simulink model "PowerPlant_Unit"  (R2021a)
settings: Solver=ode23t  StartTime=0.0  StopTime=20  RelTol=1e-3  AbsTol=1e-3
libraries: nesl_utility x15, fl_lib x13, ee_lib x9
settings Model: PacingRate=1000  Creator=ykamatan  LastModifiedBy=ykamatan
settings SolverCC: AutoScaleAbsTol=off  SolverJacobianMethodControl=SparsePerturbation  DaesscMode=Fast
settings DataIOCC: SaveOutput=off  SaveTime=off
settings DebuggingCC: SymbolicDimsDataTypeCodeGenerationDiagnostic=none  SFMachineParentedDataDiag=warning
settings SFSimCC: CustomCodeUndefinedFunction=UseInterfaceOnly
settings SimscapeCC: SimscapeLogSimulationStatistics=on  SimscapeLogDataHistory=10000

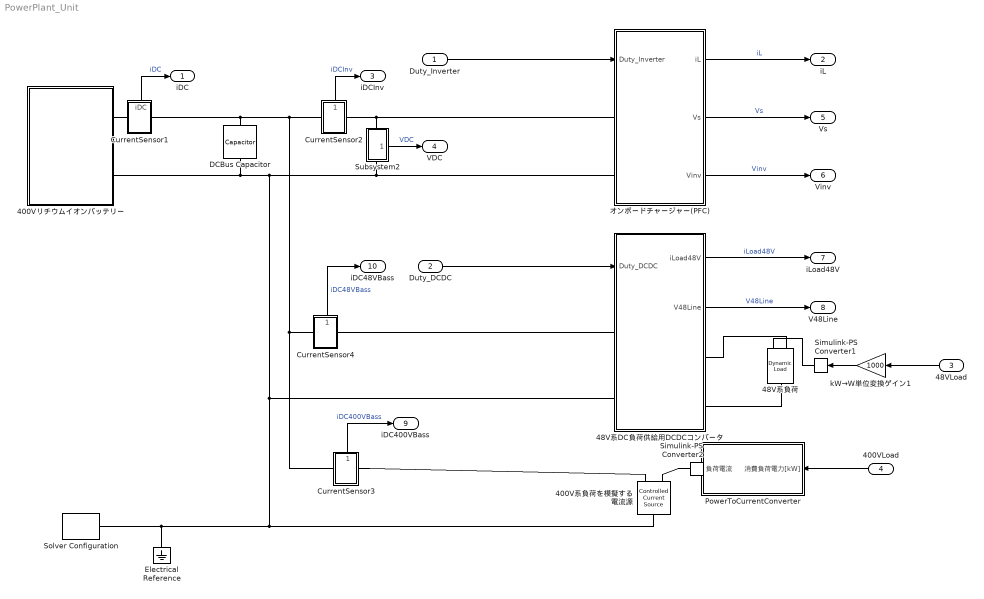
== system PowerPlant_Unit ==
  Duty_Inverter : Inport  OutDataTypeStr=double  PortDimensions=1  SampleTime=0
  Duty_DCDC : Inport  Port=2  OutDataTypeStr=double  PortDimensions=1  SampleTime=0
  48VLoad : Inport  Port=3
  400VLoad : Inport  Port=4
  400Vリチウムイオンバッテリー : Subsystem
  400V系負荷を模擬する 電流源 : fl_lib/Electrical/Electrical Sources/Controlled Current Source
  48V系DC負荷供給用DCDCコンバータ : Subsystem
  48V系負荷 : ee_lib/Passive/Dynamic Load  load_type=ee.enum.dc_ac.dc  enable_fault=ee.enum.faults.faultEnable.no  min_supply_voltage=38 V  pow_min=1e-3 W  G_reverse=1e-6 S  deltaV=1e-3 V  f0=60 Hz  Vrms_min=200 V  Pmin=1e-3 W  fault_action=ee.enum.faults.faultAction.none  t_fault=1 s  open_conductance=1e-4 S
      settings: SourceProductBaseCode=PS  InternalSimscapePortConfiguration="{\"Bottom\":[],\"Left\":[{\"id\":\"p\",\"label\":\"+\",\"type\":\"foundation.electrical.electrical\"}],\"Right\":[{\"id\":\"n\",\"label\":\"-\",\"type\":\"foundation.electrical.electrical\"}],\"Top\":[{\"id\":\"P\",\"label\":\"P\",\"type\":\"input\"}]}"
  CurrentSensor1 : Subsystem
      settings: PortSchema="{\"entries\":[{\"content\":{\"sides\":[{\"content\":{\"connectorIds\":[\"LConn1\"]},\"type\":\"ConnectorPlacement.EquallySpacedRectSide\",\"uuid\":\"7286f59e-cee0-499d-832c-cf6f33a1b017\"},{\"content\":{\"connectorIds\":[\"RConn1\"],\"side\":\"RIGHT\"},\"type\":\"ConnectorPlacement.EquallySpacedRectSide\",\"uuid\":\"6a983281-a6bc-4a57-a5ba-c4da9a8828f4\"},{\"content\":{\"connectorIds\":[\"Out1\"],\"side\":\"TOP\"},\"type\":\"ConnectorPlacement.EquallySpacedRectSide\",\"uuid\":\"6969f7e7-2dce-4d64-b6f6-e92ef9035b1a\"}]},\"type\":\"ConnectorPlacement.EquallySpacedConnector\",\"uuid\":\"05fc616a-5402-4b75-b59e-8cf259d71f3d\"}],\"packageUris\":[\"http://schema.mathworks.com/mf0/Connector/R2020b\"],\"version\":\"1.0\"}"
  CurrentSensor2 : Subsystem
      settings: PortSchema="{\"entries\":[{\"content\":{\"sides\":[{\"content\":{\"connectorIds\":[\"LConn1\"]},\"type\":\"ConnectorPlacement.EquallySpacedRectSide\",\"uuid\":\"7286f59e-cee0-499d-832c-cf6f33a1b017\"},{\"content\":{\"connectorIds\":[\"RConn1\"],\"side\":\"RIGHT\"},\"type\":\"ConnectorPlacement.EquallySpacedRectSide\",\"uuid\":\"6a983281-a6bc-4a57-a5ba-c4da9a8828f4\"},{\"content\":{\"connectorIds\":[\"Out1\"],\"side\":\"TOP\"},\"type\":\"ConnectorPlacement.EquallySpacedRectSide\",\"uuid\":\"6969f7e7-2dce-4d64-b6f6-e92ef9035b1a\"}]},\"type\":\"ConnectorPlacement.EquallySpacedConnector\",\"uuid\":\"05fc616a-5402-4b75-b59e-8cf259d71f3d\"}],\"packageUris\":[\"http://schema.mathworks.com/mf0/Connector/R2020b\"],\"version\":\"1.0\"}"
  CurrentSensor3 : Subsystem
      settings: PortSchema="{\"entries\":[{\"content\":{\"sides\":[{\"content\":{\"connectorIds\":[\"LConn1\"]},\"type\":\"ConnectorPlacement.EquallySpacedRectSide\",\"uuid\":\"7286f59e-cee0-499d-832c-cf6f33a1b017\"},{\"content\":{\"connectorIds\":[\"RConn1\"],\"side\":\"RIGHT\"},\"type\":\"ConnectorPlacement.EquallySpacedRectSide\",\"uuid\":\"6a983281-a6bc-4a57-a5ba-c4da9a8828f4\"},{\"content\":{\"connectorIds\":[\"Out1\"],\"side\":\"TOP\"},\"type\":\"ConnectorPlacement.EquallySpacedRectSide\",\"uuid\":\"6969f7e7-2dce-4d64-b6f6-e92ef9035b1a\"}]},\"type\":\"ConnectorPlacement.EquallySpacedConnector\",\"uuid\":\"05fc616a-5402-4b75-b59e-8cf259d71f3d\"}],\"packageUris\":[\"http://schema.mathworks.com/mf0/Connector/R2020b\"],\"version\":\"1.0\"}"
  CurrentSensor4 : Subsystem
      settings: PortSchema="{\"entries\":[{\"content\":{\"sides\":[{\"content\":{\"connectorIds\":[\"LConn1\"]},\"type\":\"ConnectorPlacement.EquallySpacedRectSide\",\"uuid\":\"7286f59e-cee0-499d-832c-cf6f33a1b017\"},{\"content\":{\"connectorIds\":[\"RConn1\"],\"side\":\"RIGHT\"},\"type\":\"ConnectorPlacement.EquallySpacedRectSide\",\"uuid\":\"6a983281-a6bc-4a57-a5ba-c4da9a8828f4\"},{\"content\":{\"connectorIds\":[\"Out1\"],\"side\":\"TOP\"},\"type\":\"ConnectorPlacement.EquallySpacedRectSide\",\"uuid\":\"6969f7e7-2dce-4d64-b6f6-e92ef9035b1a\"}]},\"type\":\"ConnectorPlacement.EquallySpacedConnector\",\"uuid\":\"05fc616a-5402-4b75-b59e-8cf259d71f3d\"}],\"packageUris\":[\"http://schema.mathworks.com/mf0/Connector/R2020b\"],\"version\":\"1.0\"}"
  DCBus Capacitor : ee_lib/Passive/Capacitor  cap_option=0  c=1000e-6 F  Cvec=[1e-05, 1e-06] F  Vvec=[0, 10] V  CV_table_symmetry=1  f_vec=[1, 10] kHz  DFext_vec=[.8, 1.2]  C_tol=5  enable_C_tol=0  tol_distribution=1  nSigma=4  r=1e-6 Ohm  g=0 1/Ohm  averaging_period=0 s  enable_operating_limits=0  operating_limit_action=2  max_working_voltage_range=[-25, 25] V  power_rating=1 W  enable_faults=0  fault_action=1  Cscale_faulted=100  R_faulted=1e-3 Ohm  G_faulted=0 1/Ohm  tau_fault=1e-3 s  enable_temporal_fault=0  t_fault=1 s  enable_behavioral_fault=0  max_permissible_voltage_range=[-100, 100] V  t_fail_on_voltage=1 s  i_specify=off  i_priority=None  i=0 A  i_nominal_specify=off  i_nominal_unit=A  i_nominal_value=1  v_specify=off  v_priority=None  v=400 V  v_nominal_specify=off  v_nominal_unit=V  v_nominal_value=1  vc_specify=on  vc_priority=High  vc=400 V  vc_nominal_specify=off  vc_nominal_unit=V  vc_nominal_value=1
  Electrical Reference : fl_lib/Electrical/Electrical Elements/Electrical Reference
  PowerToCurrentConverter : Subsystem
  Simulink-PS Converter1 : nesl_utility/Simulink-PS Converter  PhysicalDomain=network_engine_domain  SubClassName=ps_input  LeftPortType=input  RightPortType=output  PseudoPeriodic=off  Frequencies=[]  NoiseDistribution=none  NoiseParameters=[]  Unit=1  AffineConversion=off  FilteringAndDerivatives=provide  SimscapeFilterOrder=1  InputFilterTimeConstant=0.001  UdotUserProvided=0
      settings: SourceProductBaseCode=PW,SS
  Simulink-PS Converter2 : nesl_utility/Simulink-PS Converter  PhysicalDomain=network_engine_domain  SubClassName=ps_input  LeftPortType=input  RightPortType=output  PseudoPeriodic=off  Frequencies=[]  NoiseDistribution=none  NoiseParameters=[]  Unit=1  AffineConversion=off  FilteringAndDerivatives=provide  SimscapeFilterOrder=1  InputFilterTimeConstant=0.001  UdotUserProvided=0
      settings: SourceProductBaseCode=PW,SS
  Solver Configuration : nesl_utility/Solver Configuration  PhysicalDomain=network_engine_domain  SubClassName=solver  LeftPortType=input  RightPortType=generic  Tones=[]  Harmonics=[]  SimulateNoise=off  Profile=off  UseLocalSampling=off  EnableSwitchedLinearOptims=on  FrequencyDomain=off  UseCCode=off  RelTol=0.001  AbsTol=1e-06  MinStep=1e-09  ToWorkspace=off  RevertToSquareIcSolve=off  NumHomotopyIterations=100  PhasorMode=off  PhasorModeNumHarmonics=1  DoDC=off  ResidualTolerance=1e-09  UseLocalSolver=off  LocalSolverChoice=NE_BACKWARD_EULER_ADVANCER  LocalSolverSampleTime=0.001  DoFixedCost=off  MaxNonlinIter=3  MaxModeIter=2  ComputeImpulses=off  ImpulseIterations=2  LinearAlgebra=auto  EquationFormulation=NE_TIME_EF  DelaysMemoryBudget=1024  AutomaticFiltering=on  FilteringTimeConstant=0.001  PartitionStorageMethod=AS_NEEDED  PartitionMemoryBudget=1024  PartitionMethod=ROBUST
      settings: SourceProductBaseCode=PW,SS
  Subsystem2 : Subsystem
      settings: PortSchema="{\"entries\":[{\"content\":{\"sides\":[{\"content\":{\"connectorIds\":[\"Out1\"]},\"type\":\"ConnectorPlacement.EquallySpacedRectSide\",\"uuid\":\"7286f59e-cee0-499d-832c-cf6f33a1b017\"},{\"content\":{\"connectorIds\":[],\"side\":\"RIGHT\"},\"type\":\"ConnectorPlacement.EquallySpacedRectSide\",\"uuid\":\"6a983281-a6bc-4a57-a5ba-c4da9a8828f4\"},{\"content\":{\"connectorIds\":[\"LConn1\"],\"side\":\"TOP\"},\"type\":\"ConnectorPlacement.EquallySpacedRectSide\",\"uuid\":\"6969f7e7-2dce-4d64-b6f6-e92ef9035b1a\"},{\"content\":{\"connectorIds\":[\"RConn1\"],\"side\":\"BOTTOM\"},\"type\":\"ConnectorPlacement.EquallySpacedRectSide\",\"uuid\":\"8f7d22cd-967a-487e-912d-7270502758f1\"}]},\"type\":\"ConnectorPlacement.EquallySpacedConnector\",\"uuid\":\"05fc616a-5402-4b75-b59e-8cf259d71f3d\"}],\"packageUris\":[\"http://schema.mathworks.com/mf0/Connector/R2020b\"],\"version\":\"1.0\"}"
  kW→W単位変換ゲイン1 : Gain  Gain=1000
  オンボードチャージャー(PFC) : Subsystem
  iDC : Outport  OutDataTypeStr=double  PortDimensions=1  SampleTime=0
  iL : Outport  Port=2  OutDataTypeStr=double  PortDimensions=1  SampleTime=0
  iDCInv : Outport  Port=3  OutDataTypeStr=double  PortDimensions=1  SampleTime=0
  VDC : Outport  Port=4  OutDataTypeStr=double  PortDimensions=1  SampleTime=0
  Vs : Outport  Port=5  OutDataTypeStr=double  PortDimensions=1  SampleTime=0
  Vinv : Outport  Port=6  OutDataTypeStr=double  PortDimensions=1  SampleTime=0
  iLoad48V : Outport  Port=7  OutDataTypeStr=double  PortDimensions=1  SampleTime=0
  V48Line : Outport  Port=8  OutDataTypeStr=double  PortDimensions=1  SampleTime=0
  iDC400VBass : Outport  Port=9  OutDataTypeStr=double  PortDimensions=1  SampleTime=0
  iDC48VBass : Outport  Port=10  OutDataTypeStr=double  PortDimensions=1  SampleTime=0
  wires:
  48V系DC負荷供給用DCDCコンバータ/1(iLoad48V) -> iLoad48V/1  "iLoad48V"
  オンボードチャージャー(PFC)/3(Vinv) -> Vinv/1  "Vinv"
  CurrentSensor2/1(iDCInv) -> iDCInv/1  "iDCInv"
  48V系DC負荷供給用DCDCコンバータ/2(V48Line) -> V48Line/1  "V48Line"
  CurrentSensor1/1(iDC) -> iDC/1  "iDC"
  オンボードチャージャー(PFC)/2(Vs) -> Vs/1  "Vs"
  PowerToCurrentConverter/1(負荷電流) -> Simulink-PS Converter2/1
  400VLoad/1 -> PowerToCurrentConverter/1(消費負荷電力[kW])
  CurrentSensor3/1(iDC400VBass) -> iDC400VBass/1  "iDC400VBass"
  kW→W単位変換ゲイン1/1 -> Simulink-PS Converter1/1
  48VLoad/1 -> kW→W単位変換ゲイン1/1
  Subsystem2/1(Vdc) -> VDC/1  "VDC"
  Duty_Inverter/1 -> オンボードチャージャー(PFC)/1(Duty_Inverter)
  CurrentSensor4/1(iDC48VBass) -> iDC48VBass/1  "iDC48VBass"
  オンボードチャージャー(PFC)/1(iL) -> iL/1  "iL"
  Duty_DCDC/1 -> 48V系DC負荷供給用DCDCコンバータ/1(Duty_DCDC)
  connections:
  400Vリチウムイオンバッテリー/RConn2 -- DCBus Capacitor/RConn1 -- Solver Configuration/RConn1 -- Electrical Reference/LConn1 -- 400V系負荷を模擬する 電流源/LConn1 -- 48V系DC負荷供給用DCDCコンバータ/LConn2 -- Subsystem2/RConn1 -- オンボードチャージャー(PFC)/LConn2
  Subsystem2/LConn1 -- CurrentSensor2/RConn1 -- オンボードチャージャー(PFC)/LConn1
  CurrentSensor2/LConn1 -- CurrentSensor3/LConn1 -- CurrentSensor4/LConn1 -- DCBus Capacitor/LConn1 -- CurrentSensor1/RConn1
  Simulink-PS Converter2/RConn1 -- 400V系負荷を模擬する 電流源/RConn1
  CurrentSensor1/LConn1 -- 400Vリチウムイオンバッテリー/RConn1
  48V系負荷/RConn1 -- 48V系DC負荷供給用DCDCコンバータ/RConn2
  48V系DC負荷供給用DCDCコンバータ/RConn1 -- 48V系負荷/LConn1
  Simulink-PS Converter1/RConn1 -- 48V系負荷/LConn2
  CurrentSensor3/RConn1 -- 400V系負荷を模擬する 電流源/RConn2
  CurrentSensor4/RConn1 -- 48V系DC負荷供給用DCDCコンバータ/LConn1

== system PowerPlant_Unit/400Vリチウムイオンバッテリー ==
  400V 理想特性蓄電池 : ee_lib/Sources/Battery  Vnom=400 V  prm_dir=1  R1_dis=2 Ohm  R1_ch=2 Ohm  R1=1 Ohm  prm_AH=2  AH=0.5 hr*A  V1=380 V  AH1=0.25 hr*A  prm_R2=1  R2=2000 Ohm  prm_dyn=2  Rp1=0.05 Ohm  tau1=30 s  Rp2=0.005 Ohm  tau2=30 s  Rp3=0.005 Ohm  tau3=30 s  Rp4=0.005 Ohm  tau4=30 s  Rp5=0.005 Ohm  tau5=30 s  prm_fade=1  N_fade=100  AH_fade=45 hr*A  R1_fade=2.02 Ohm  R1_ch_fade=2.02 Ohm  V1_fade=10.35 V  prm_age=1  prm_age_OCV=1  OCV_age=0.9  SOC_age=60  Tmeas_age=298.15 K  delta_time_age_vec=[0] d  temperature_age_vec=[273] K  OCV_scaling_age=2.2134e6  OCV_offset_age=1.632e6  temp_exp_age=0.515833569 V  t_exp_age=0.75  i_specify=off  i_priority=None  i=0 A  i_nominal_specify=off  i_nominal_unit=A  i_nominal_value=1  v_specify=off  v_priority=None  v=0 V  v_nominal_specify=off  v_nominal_unit=V  v_nominal_value=1  charge_specify=on  charge_priority=High  charge=0.25 hr*A  charge_nominal_specify=off  charge_nominal_unit=hr*A  charge_nominal_value=1  num_cycles_specify=off  num_cycles_priority=High  num_cycles=0  num_cycles_nominal_specify=off  num_cycles_nominal_unit=1  num_cycles_nominal_value=1  thermal_mass=30000 J/K  Tmeas=298.15 K  Vnom_T2=12 V  R1_T2=2.2 Ohm  R1_T2_dis=2.2 Ohm  R1_T2_ch=2.2 Ohm  V1_T2=11.4 V  R2_T2=2200 Ohm  Rp1_T2=0.005 Ohm  tau1_T2=30 s  Rp2_T2=0.005 Ohm  tau2_T2=30 s  Rp3_T2=0.005 Ohm  tau3_T2=30 s  Rp4_T2=0.005 Ohm  tau4_T2=30 s  Rp5_T2=0.005 Ohm  tau5_T2=30 s  Tmeas2=273.15 K  temperature_specify=off  temperature_priority=High  temperature=298.15 K  temperature_nominal_specify=off  temperature_nominal_unit=K  temperature_nominal_value=1
  Bat+ : PMIOPort  Side=Right
  Bat- : PMIOPort  Port=2  Side=Right
  connections:
  400V 理想特性蓄電池/RConn1 -- Bat-/RConn1
  Bat+/RConn1 -- 400V 理想特性蓄電池/LConn1

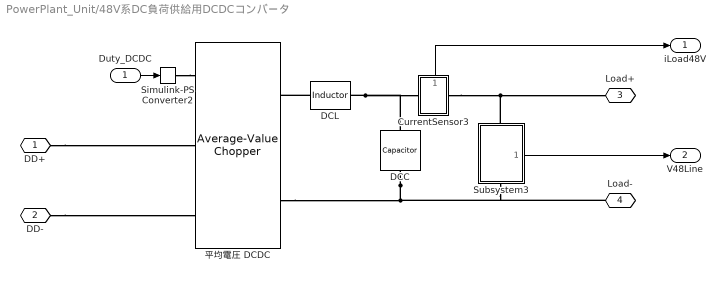
== system PowerPlant_Unit/48V系DC負荷供給用DCDCコンバータ ==
  Duty_DCDC : Inport
  CurrentSensor3 : Subsystem
      settings: PortSchema="{\"entries\":[{\"content\":{\"sides\":[{\"content\":{\"connectorIds\":[\"LConn1\"]},\"type\":\"ConnectorPlacement.EquallySpacedRectSide\",\"uuid\":\"7286f59e-cee0-499d-832c-cf6f33a1b017\"},{\"content\":{\"connectorIds\":[\"RConn1\"],\"side\":\"RIGHT\"},\"type\":\"ConnectorPlacement.EquallySpacedRectSide\",\"uuid\":\"6a983281-a6bc-4a57-a5ba-c4da9a8828f4\"},{\"content\":{\"connectorIds\":[\"Out1\"],\"side\":\"TOP\"},\"type\":\"ConnectorPlacement.EquallySpacedRectSide\",\"uuid\":\"6969f7e7-2dce-4d64-b6f6-e92ef9035b1a\"}]},\"type\":\"ConnectorPlacement.EquallySpacedConnector\",\"uuid\":\"05fc616a-5402-4b75-b59e-8cf259d71f3d\"}],\"packageUris\":[\"http://schema.mathworks.com/mf0/Connector/R2020b\"],\"version\":\"1.0\"}"
  DCC : ee_lib/Passive/Capacitor  cap_option=0  c=100e-6 F  Cvec=[1e-05, 1e-06] F  Vvec=[0, 10] V  CV_table_symmetry=1  f_vec=[1, 10] kHz  DFext_vec=[.8, 1.2]  C_tol=5  enable_C_tol=0  tol_distribution=1  nSigma=4  r=100e-3 Ohm  g=0 1/Ohm  averaging_period=0 s  enable_operating_limits=0  operating_limit_action=2  max_working_voltage_range=[-25, 25] V  power_rating=1 W  enable_faults=0  fault_action=1  Cscale_faulted=100  R_faulted=1e-3 Ohm  G_faulted=0 1/Ohm  tau_fault=1e-3 s  enable_temporal_fault=0  t_fault=1 s  enable_behavioral_fault=0  max_permissible_voltage_range=[-100, 100] V  t_fail_on_voltage=1 s  i_specify=off  i_priority=None  i=0 A  i_nominal_specify=off  i_nominal_unit=A  i_nominal_value=1  v_specify=off  v_priority=None  v=400 V  v_nominal_specify=off  v_nominal_unit=V  v_nominal_value=1  vc_specify=on  vc_priority=High  vc=48 V  vc_nominal_specify=off  vc_nominal_unit=V  vc_nominal_value=1
  DCL : ee_lib/Passive/Inductor  l=10e-6 H  L_tol=20  enable_L_tol=0  tol_distribution=1  nSigma=4  r=0.1 Ohm  g=1e-9 1/Ohm  enable_operating_limits=0  operating_limit_action=2  max_working_current=1 A  power_rating=1 W  enable_faults=0  fault_action=1  lambdaPercent=50  k_faulted=0.9999  turnsShort=0  openCct=0  groundShort=0  groundShortG=0 1/Ohm  tau_fault=1e-3 s  enable_temporal_fault=0  t_fault=1 s  enable_behavioral_fault=0  max_permissible_voltage=100 V  n_fail_on_voltage=1  max_permissible_current=1 A  t_fail_on_current=1 s  i_L_specify=off  i_L_priority=High  i_L=0 A  i_L_nominal_specify=off  i_L_nominal_unit=A  i_L_nominal_value=1
  Simulink-PS Converter2 : nesl_utility/Simulink-PS Converter  PhysicalDomain=network_engine_domain  SubClassName=ps_input  LeftPortType=input  RightPortType=output  PseudoPeriodic=off  Frequencies=[]  NoiseDistribution=none  NoiseParameters=[]  Unit=1  AffineConversion=off  FilteringAndDerivatives=provide  SimscapeFilterOrder=1  InputFilterTimeConstant=0.001  UdotUserProvided=0
      settings: SourceProductBaseCode=PW,SS
  Subsystem3 : Subsystem
      settings: PortSchema="{\"entries\":[{\"content\":{\"sides\":[{\"content\":{\"connectorIds\":[]},\"type\":\"ConnectorPlacement.EquallySpacedRectSide\",\"uuid\":\"7286f59e-cee0-499d-832c-cf6f33a1b017\"},{\"content\":{\"connectorIds\":[\"Out1\"],\"side\":\"RIGHT\"},\"type\":\"ConnectorPlacement.EquallySpacedRectSide\",\"uuid\":\"6a983281-a6bc-4a57-a5ba-c4da9a8828f4\"},{\"content\":{\"connectorIds\":[\"LConn1\"],\"side\":\"TOP\"},\"type\":\"ConnectorPlacement.EquallySpacedRectSide\",\"uuid\":\"6969f7e7-2dce-4d64-b6f6-e92ef9035b1a\"},{\"content\":{\"connectorIds\":[\"RConn1\"],\"side\":\"BOTTOM\"},\"type\":\"ConnectorPlacement.EquallySpacedRectSide\",\"uuid\":\"8f7d22cd-967a-487e-912d-7270502758f1\"}]},\"type\":\"ConnectorPlacement.EquallySpacedConnector\",\"uuid\":\"05fc616a-5402-4b75-b59e-8cf259d71f3d\"}],\"packageUris\":[\"http://schema.mathworks.com/mf0/Connector/R2020b\"],\"version\":\"1.0\"}"
  平均電圧 DCDC : ee_lib/Semiconductors & Converters/Converters/Average-Value Chopper  chopper_type=5  efficiency_option=1  efficiency_fixed=100  i_vec=[0, 2, 5] A  efficiency_vec=[90, 95, 98]
      settings: SourceProductBaseCode=PS  InternalSimscapePortConfiguration="{\"Bottom\":[],\"Left\":[{\"id\":\"DutyCycle\",\"label\":\"DutyCycle\",\"type\":\"input\"},{\"id\":\"p1\",\"label\":\"1+\",\"type\":\"foundation.electrical.electrical\"},{\"id\":\"n1\",\"label\":\"1-\",\"type\":\"foundation.electrical.electrical\"}],\"Right\":[{\"id\":\"p2\",\"label\":\"2+\",\"type\":\"foundation.electrical.electrical\"},{\"id\":\"n2\",\"label\":\"2-\",\"type\":\"foundation.electrical.electrical\"}],\"Top\":[]}"
  DD+ : PMIOPort  Side=Left
  DD- : PMIOPort  Port=2  Side=Left
  Load+ : PMIOPort  Port=3  Side=Right
  Load- : PMIOPort  Port=4  Side=Right
  iLoad48V : Outport
  V48Line : Outport  Port=2
  wires:
  CurrentSensor3/1(iLoad48V) -> iLoad48V/1
  Subsystem3/1(V48Line) -> V48Line/1
  Duty_DCDC/1 -> Simulink-PS Converter2/1
  connections:
  DD+/RConn1 -- 平均電圧 DCDC/LConn2
  CurrentSensor3/RConn1 -- Load+/RConn1 -- Subsystem3/LConn1
  DCL/LConn1 -- 平均電圧 DCDC/RConn1
  DCL/RConn1 -- CurrentSensor3/LConn1 -- DCC/LConn1
  DD-/RConn1 -- 平均電圧 DCDC/LConn3
  DCC/RConn1 -- Load-/RConn1 -- Subsystem3/RConn1 -- 平均電圧 DCDC/RConn2
  Simulink-PS Converter2/RConn1 -- 平均電圧 DCDC/LConn1

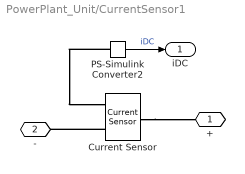
== system PowerPlant_Unit/CurrentSensor1 ==
  Current Sensor : fl_lib/Electrical/Electrical Sensors/Current Sensor
  PS-Simulink Converter2 : nesl_utility/PS-Simulink Converter  PhysicalDomain=network_engine_domain  SubClassName=ps_output  LeftPortType=input  RightPortType=output  PseudoPeriodic=off  Frequencies=[]  Unit=inherit  AffineConversion=off
      settings: SourceProductBaseCode=PW,SS
  + : PMIOPort  Side=Left
  - : PMIOPort  Port=2  Side=Right
  iDC : Outport
  wires:
  PS-Simulink Converter2/1 -> iDC/1  "iDC"
  connections:
  Current Sensor/RConn2 -- -/RConn1
  PS-Simulink Converter2/LConn1 -- Current Sensor/RConn1
  Current Sensor/LConn1 -- +/RConn1

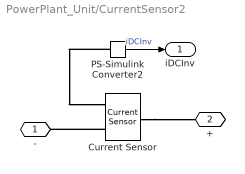
== system PowerPlant_Unit/CurrentSensor2 ==
  Current Sensor : fl_lib/Electrical/Electrical Sensors/Current Sensor
  PS-Simulink Converter2 : nesl_utility/PS-Simulink Converter  PhysicalDomain=network_engine_domain  SubClassName=ps_output  LeftPortType=input  RightPortType=output  PseudoPeriodic=off  Frequencies=[]  Unit=inherit  AffineConversion=off
      settings: SourceProductBaseCode=PW,SS
  - : PMIOPort  Side=Left
  + : PMIOPort  Port=2  Side=Right
  iDCInv : Outport
  wires:
  PS-Simulink Converter2/1 -> iDCInv/1  "iDCInv"
  connections:
  Current Sensor/RConn2 -- -/RConn1
  PS-Simulink Converter2/LConn1 -- Current Sensor/RConn1
  Current Sensor/LConn1 -- +/RConn1

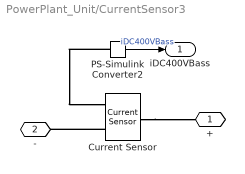
== system PowerPlant_Unit/CurrentSensor3 ==
  Current Sensor : fl_lib/Electrical/Electrical Sensors/Current Sensor
  PS-Simulink Converter2 : nesl_utility/PS-Simulink Converter  PhysicalDomain=network_engine_domain  SubClassName=ps_output  LeftPortType=input  RightPortType=output  PseudoPeriodic=off  Frequencies=[]  Unit=inherit  AffineConversion=off
      settings: SourceProductBaseCode=PW,SS
  + : PMIOPort  Side=Left
  - : PMIOPort  Port=2  Side=Right
  iDC400VBass : Outport
  wires:
  PS-Simulink Converter2/1 -> iDC400VBass/1  "iDC400VBass"
  connections:
  Current Sensor/RConn2 -- -/RConn1
  PS-Simulink Converter2/LConn1 -- Current Sensor/RConn1
  Current Sensor/LConn1 -- +/RConn1

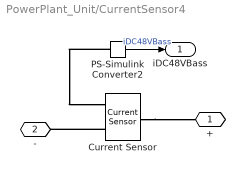
== system PowerPlant_Unit/CurrentSensor4 ==
  Current Sensor : fl_lib/Electrical/Electrical Sensors/Current Sensor
  PS-Simulink Converter2 : nesl_utility/PS-Simulink Converter  PhysicalDomain=network_engine_domain  SubClassName=ps_output  LeftPortType=input  RightPortType=output  PseudoPeriodic=off  Frequencies=[]  Unit=inherit  AffineConversion=off
      settings: SourceProductBaseCode=PW,SS
  + : PMIOPort  Side=Left
  - : PMIOPort  Port=2  Side=Right
  iDC48VBass : Outport
  wires:
  PS-Simulink Converter2/1 -> iDC48VBass/1  "iDC48VBass"
  connections:
  Current Sensor/RConn2 -- -/RConn1
  PS-Simulink Converter2/LConn1 -- Current Sensor/RConn1
  Current Sensor/LConn1 -- +/RConn1

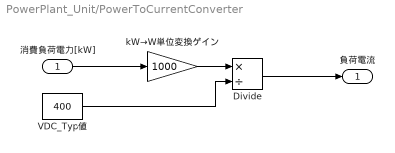
== system PowerPlant_Unit/PowerToCurrentConverter ==
  消費負荷電力[kW] : Inport
  Divide : Product  Inputs=*/
  VDC_Typ値 : Constant  Value=400
  kW→W単位変換ゲイン : Gain  Gain=1000
  負荷電流 : Outport
  wires:
  Divide/1 -> 負荷電流/1
  VDC_Typ値/1 -> Divide/2
  kW→W単位変換ゲイン/1 -> Divide/1
  消費負荷電力[kW]/1 -> kW→W単位変換ゲイン/1

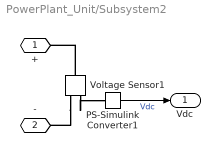
== system PowerPlant_Unit/Subsystem2 ==
  PS-Simulink Converter1 : nesl_utility/PS-Simulink Converter  PhysicalDomain=network_engine_domain  SubClassName=ps_output  LeftPortType=input  RightPortType=output  PseudoPeriodic=off  Frequencies=[]  Unit=inherit  AffineConversion=off
      settings: SourceProductBaseCode=PW,SS
  Voltage Sensor1 : fl_lib/Electrical/Electrical Sensors/Voltage Sensor
  + : PMIOPort  Side=Left
  - : PMIOPort  Port=2  Side=Right
  Vdc : Outport
  wires:
  PS-Simulink Converter1/1 -> Vdc/1  "Vdc"
  connections:
  Voltage Sensor1/RConn2 -- -/RConn1
  Voltage Sensor1/LConn1 -- +/RConn1
  Voltage Sensor1/RConn1 -- PS-Simulink Converter1/LConn1

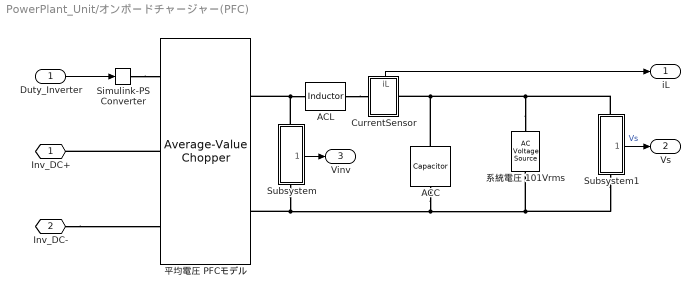
== system PowerPlant_Unit/オンボードチャージャー(PFC) ==
  Duty_Inverter : Inport
  ACC : ee_lib/Passive/Capacitor  cap_option=0  c=10e-6 F  Cvec=[1e-05, 1e-06] F  Vvec=[0, 10] V  CV_table_symmetry=1  f_vec=[1, 10] kHz  DFext_vec=[.8, 1.2]  C_tol=5  enable_C_tol=0  tol_distribution=1  nSigma=4  r=100e-3 Ohm  g=0 1/Ohm  averaging_period=0 s  enable_operating_limits=0  operating_limit_action=2  max_working_voltage_range=[-25, 25] V  power_rating=1 W  enable_faults=0  fault_action=1  Cscale_faulted=100  R_faulted=1e-3 Ohm  G_faulted=0 1/Ohm  tau_fault=1e-3 s  enable_temporal_fault=0  t_fault=1 s  enable_behavioral_fault=0  max_permissible_voltage_range=[-100, 100] V  t_fail_on_voltage=1 s  i_specify=off  i_priority=None  i=0 A  i_nominal_specify=off  i_nominal_unit=A  i_nominal_value=1  v_specify=off  v_priority=None  v=400 V  v_nominal_specify=off  v_nominal_unit=V  v_nominal_value=1  vc_specify=off  vc_priority=High  vc=48 V  vc_nominal_specify=off  vc_nominal_unit=V  vc_nominal_value=1
  ACL : ee_lib/Passive/Inductor  l=1e-3 H  L_tol=20  enable_L_tol=0  tol_distribution=1  nSigma=4  r=0.1 Ohm  g=1e-9 1/Ohm  enable_operating_limits=0  operating_limit_action=2  max_working_current=1 A  power_rating=1 W  enable_faults=0  fault_action=1  lambdaPercent=50  k_faulted=0.9999  turnsShort=0  openCct=0  groundShort=0  groundShortG=0 1/Ohm  tau_fault=1e-3 s  enable_temporal_fault=0  t_fault=1 s  enable_behavioral_fault=0  max_permissible_voltage=100 V  n_fail_on_voltage=1  max_permissible_current=1 A  t_fail_on_current=1 s  i_L_specify=off  i_L_priority=High  i_L=0 A  i_L_nominal_specify=off  i_L_nominal_unit=A  i_L_nominal_value=1
  CurrentSensor : Subsystem
      settings: PortSchema="{\"entries\":[{\"content\":{\"sides\":[{\"content\":{\"connectorIds\":[\"LConn1\"]},\"type\":\"ConnectorPlacement.EquallySpacedRectSide\",\"uuid\":\"7286f59e-cee0-499d-832c-cf6f33a1b017\"},{\"content\":{\"connectorIds\":[\"RConn1\"],\"side\":\"RIGHT\"},\"type\":\"ConnectorPlacement.EquallySpacedRectSide\",\"uuid\":\"6a983281-a6bc-4a57-a5ba-c4da9a8828f4\"},{\"content\":{\"connectorIds\":[\"Out1\"],\"side\":\"TOP\"},\"type\":\"ConnectorPlacement.EquallySpacedRectSide\",\"uuid\":\"6969f7e7-2dce-4d64-b6f6-e92ef9035b1a\"}]},\"type\":\"ConnectorPlacement.EquallySpacedConnector\",\"uuid\":\"05fc616a-5402-4b75-b59e-8cf259d71f3d\"}],\"packageUris\":[\"http://schema.mathworks.com/mf0/Connector/R2020b\"],\"version\":\"1.0\"}"
  Simulink-PS Converter : nesl_utility/Simulink-PS Converter  PhysicalDomain=network_engine_domain  SubClassName=ps_input  LeftPortType=input  RightPortType=output  PseudoPeriodic=off  Frequencies=[]  NoiseDistribution=none  NoiseParameters=[]  Unit=1  AffineConversion=off  FilteringAndDerivatives=provide  SimscapeFilterOrder=1  InputFilterTimeConstant=0.001  UdotUserProvided=0
      settings: SourceProductBaseCode=PW,SS
  Subsystem : Subsystem
      settings: PortSchema="{\"entries\":[{\"content\":{\"sides\":[{\"content\":{\"connectorIds\":[]},\"type\":\"ConnectorPlacement.EquallySpacedRectSide\",\"uuid\":\"7286f59e-cee0-499d-832c-cf6f33a1b017\"},{\"content\":{\"connectorIds\":[\"Out1\"],\"side\":\"RIGHT\"},\"type\":\"ConnectorPlacement.EquallySpacedRectSide\",\"uuid\":\"6a983281-a6bc-4a57-a5ba-c4da9a8828f4\"},{\"content\":{\"connectorIds\":[\"LConn1\"],\"side\":\"TOP\"},\"type\":\"ConnectorPlacement.EquallySpacedRectSide\",\"uuid\":\"6969f7e7-2dce-4d64-b6f6-e92ef9035b1a\"},{\"content\":{\"connectorIds\":[\"RConn1\"],\"side\":\"BOTTOM\"},\"type\":\"ConnectorPlacement.EquallySpacedRectSide\",\"uuid\":\"8f7d22cd-967a-487e-912d-7270502758f1\"}]},\"type\":\"ConnectorPlacement.EquallySpacedConnector\",\"uuid\":\"05fc616a-5402-4b75-b59e-8cf259d71f3d\"}],\"packageUris\":[\"http://schema.mathworks.com/mf0/Connector/R2020b\"],\"version\":\"1.0\"}"
  Subsystem1 : Subsystem
      settings: PortSchema="{\"entries\":[{\"content\":{\"sides\":[{\"content\":{\"connectorIds\":[]},\"type\":\"ConnectorPlacement.EquallySpacedRectSide\",\"uuid\":\"7286f59e-cee0-499d-832c-cf6f33a1b017\"},{\"content\":{\"connectorIds\":[\"Out1\"],\"side\":\"RIGHT\"},\"type\":\"ConnectorPlacement.EquallySpacedRectSide\",\"uuid\":\"6a983281-a6bc-4a57-a5ba-c4da9a8828f4\"},{\"content\":{\"connectorIds\":[\"LConn1\"],\"side\":\"TOP\"},\"type\":\"ConnectorPlacement.EquallySpacedRectSide\",\"uuid\":\"6969f7e7-2dce-4d64-b6f6-e92ef9035b1a\"},{\"content\":{\"connectorIds\":[\"RConn1\"],\"side\":\"BOTTOM\"},\"type\":\"ConnectorPlacement.EquallySpacedRectSide\",\"uuid\":\"8f7d22cd-967a-487e-912d-7270502758f1\"}]},\"type\":\"ConnectorPlacement.EquallySpacedConnector\",\"uuid\":\"05fc616a-5402-4b75-b59e-8cf259d71f3d\"}],\"packageUris\":[\"http://schema.mathworks.com/mf0/Connector/R2020b\"],\"version\":\"1.0\"}"
  平均電圧 PFCモデル : ee_lib/Semiconductors & Converters/Converters/Average-Value Chopper  chopper_type=5  efficiency_option=1  efficiency_fixed=100  i_vec=[0, 2, 5] A  efficiency_vec=[90, 95, 98]
      settings: SourceProductBaseCode=PS  InternalSimscapePortConfiguration="{\"Bottom\":[],\"Left\":[{\"id\":\"DutyCycle\",\"label\":\"DutyCycle\",\"type\":\"input\"},{\"id\":\"p1\",\"label\":\"1+\",\"type\":\"foundation.electrical.electrical\"},{\"id\":\"n1\",\"label\":\"1-\",\"type\":\"foundation.electrical.electrical\"}],\"Right\":[{\"id\":\"p2\",\"label\":\"2+\",\"type\":\"foundation.electrical.electrical\"},{\"id\":\"n2\",\"label\":\"2-\",\"type\":\"foundation.electrical.electrical\"}],\"Top\":[]}"
  系統電圧 101Vrms : fl_lib/Electrical/Electrical Sources/AC Voltage Source  amp=101*1.414 V  shift=0 deg  frequency=60 Hz  omega=0 rad/s
  Inv_DC+ : PMIOPort  Side=Left
  Inv_DC- : PMIOPort  Port=2  Side=Left
  iL : Outport
  Vs : Outport  Port=2
  Vinv : Outport  Port=3
  wires:
  Subsystem1/1(Vs) -> Vs/1  "Vs"
  Subsystem/1(Vinv) -> Vinv/1
  CurrentSensor/1(iL) -> iL/1
  Duty_Inverter/1 -> Simulink-PS Converter/1
  connections:
  平均電圧 PFCモデル/LConn2 -- Inv_DC+/RConn1
  Inv_DC-/RConn1 -- 平均電圧 PFCモデル/LConn3
  Simulink-PS Converter/RConn1 -- 平均電圧 PFCモデル/LConn1
  系統電圧 101Vrms/LConn1 -- CurrentSensor/RConn1 -- ACC/LConn1 -- Subsystem1/LConn1
  ACL/LConn1 -- 平均電圧 PFCモデル/RConn1 -- Subsystem/LConn1
  系統電圧 101Vrms/RConn1 -- Subsystem/RConn1 -- 平均電圧 PFCモデル/RConn2 -- ACC/RConn1 -- Subsystem1/RConn1
  ACL/RConn1 -- CurrentSensor/LConn1

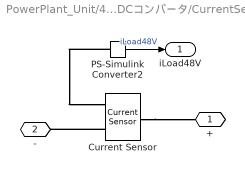
== system PowerPlant_Unit/48V系DC負荷供給用DCDCコンバータ/CurrentSensor3 ==
  Current Sensor : fl_lib/Electrical/Electrical Sensors/Current Sensor
  PS-Simulink Converter2 : nesl_utility/PS-Simulink Converter  PhysicalDomain=network_engine_domain  SubClassName=ps_output  LeftPortType=input  RightPortType=output  PseudoPeriodic=off  Frequencies=[]  Unit=inherit  AffineConversion=off
      settings: SourceProductBaseCode=PW,SS
  + : PMIOPort  Side=Left
  - : PMIOPort  Port=2  Side=Right
  iLoad48V : Outport
  wires:
  PS-Simulink Converter2/1 -> iLoad48V/1  "iLoad48V"
  connections:
  Current Sensor/RConn2 -- -/RConn1
  PS-Simulink Converter2/LConn1 -- Current Sensor/RConn1
  Current Sensor/LConn1 -- +/RConn1

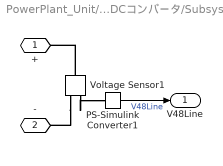
== system PowerPlant_Unit/48V系DC負荷供給用DCDCコンバータ/Subsystem3 ==
  PS-Simulink Converter1 : nesl_utility/PS-Simulink Converter  PhysicalDomain=network_engine_domain  SubClassName=ps_output  LeftPortType=input  RightPortType=output  PseudoPeriodic=off  Frequencies=[]  Unit=inherit  AffineConversion=off
      settings: SourceProductBaseCode=PW,SS
  Voltage Sensor1 : fl_lib/Electrical/Electrical Sensors/Voltage Sensor
  + : PMIOPort  Side=Left
  - : PMIOPort  Port=2  Side=Right
  V48Line : Outport
  wires:
  PS-Simulink Converter1/1 -> V48Line/1  "V48Line"
  connections:
  Voltage Sensor1/RConn2 -- -/RConn1
  Voltage Sensor1/LConn1 -- +/RConn1
  Voltage Sensor1/RConn1 -- PS-Simulink Converter1/LConn1

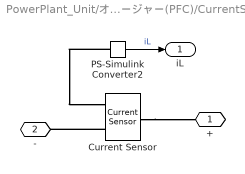
== system PowerPlant_Unit/オンボードチャージャー(PFC)/CurrentSensor ==
  Current Sensor : fl_lib/Electrical/Electrical Sensors/Current Sensor
  PS-Simulink Converter2 : nesl_utility/PS-Simulink Converter  PhysicalDomain=network_engine_domain  SubClassName=ps_output  LeftPortType=input  RightPortType=output  PseudoPeriodic=off  Frequencies=[]  Unit=inherit  AffineConversion=off
      settings: SourceProductBaseCode=PW,SS
  + : PMIOPort  Side=Left
  - : PMIOPort  Port=2  Side=Right
  iL : Outport
  wires:
  PS-Simulink Converter2/1 -> iL/1  "iL"
  connections:
  Current Sensor/RConn2 -- -/RConn1
  PS-Simulink Converter2/LConn1 -- Current Sensor/RConn1
  Current Sensor/LConn1 -- +/RConn1

== system PowerPlant_Unit/オンボードチャージャー(PFC)/Subsystem ==
  PS-Simulink Converter1 : nesl_utility/PS-Simulink Converter  PhysicalDomain=network_engine_domain  SubClassName=ps_output  LeftPortType=input  RightPortType=output  PseudoPeriodic=off  Frequencies=[]  Unit=inherit  AffineConversion=off
      settings: SourceProductBaseCode=PW,SS
  Voltage Sensor1 : fl_lib/Electrical/Electrical Sensors/Voltage Sensor
  + : PMIOPort  Side=Left
  - : PMIOPort  Port=2  Side=Right
  Vinv : Outport
  wires:
  PS-Simulink Converter1/1 -> Vinv/1  "Vinv"
  connections:
  Voltage Sensor1/RConn2 -- -/RConn1
  Voltage Sensor1/LConn1 -- +/RConn1
  Voltage Sensor1/RConn1 -- PS-Simulink Converter1/LConn1

== system PowerPlant_Unit/オンボードチャージャー(PFC)/Subsystem1 ==
  PS-Simulink Converter1 : nesl_utility/PS-Simulink Converter  PhysicalDomain=network_engine_domain  SubClassName=ps_output  LeftPortType=input  RightPortType=output  PseudoPeriodic=off  Frequencies=[]  Unit=inherit  AffineConversion=off
      settings: SourceProductBaseCode=PW,SS
  Voltage Sensor1 : fl_lib/Electrical/Electrical Sensors/Voltage Sensor
  + : PMIOPort  Side=Left
  - : PMIOPort  Port=2  Side=Right
  Vs : Outport
  wires:
  PS-Simulink Converter1/1 -> Vs/1  "Vs"
  connections:
  Voltage Sensor1/RConn2 -- -/RConn1
  Voltage Sensor1/LConn1 -- +/RConn1
  Voltage Sensor1/RConn1 -- PS-Simulink Converter1/LConn1
